simulink model "BlueBird_Formation"  (R2014a)
settings: Solver=FixedStepDiscrete  StartTime=0.0  StopTime=inf  FixedStep=0.033  RelTol=1e-3
undefined symbols (not defined in the file or in its folder): BlueBird_uni_todiff, simiam, Z_Ref
libraries: KSim x4
settings Model: SnapshotBufferSize=100  Creator=jdelacroix  LastModifiedBy=Bird
settings DataIOCC: SignalLoggingSaveFormat=ModelDataLogs
settings OptimizationCC: ExpressionDepthLimit=2147483647
settings DebuggingCC: UnderspecifiedInitializationDetection=Classic  FcnCallInpInsideContextMsg=EnableAllAsWarning  StateNameClashWarn=warning

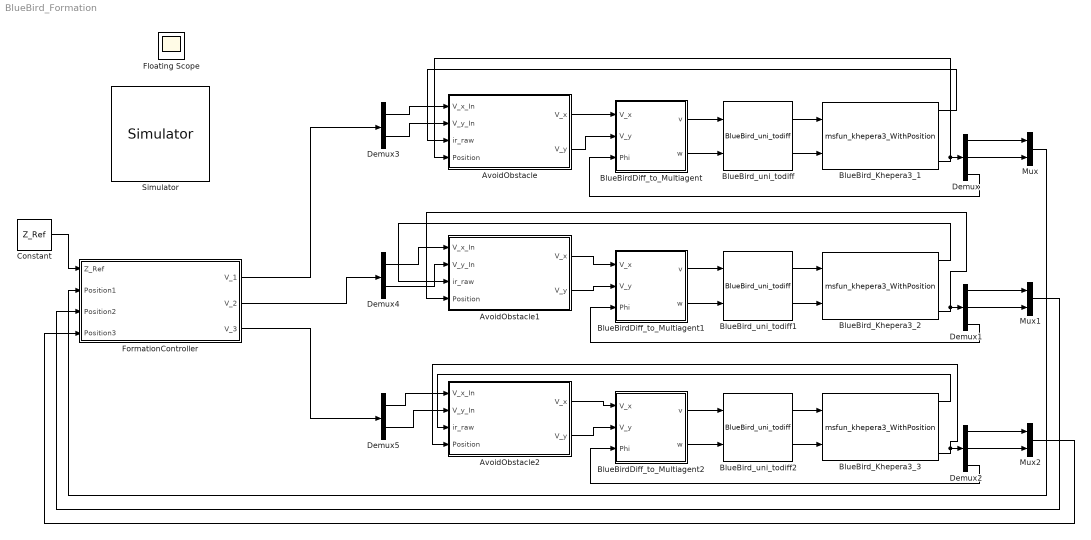
== system BlueBird_Formation ==
  AvoidObstacle : MATLAB Function  TreatAsAtomicUnit=on
  AvoidObstacle1 : MATLAB Function  TreatAsAtomicUnit=on
  AvoidObstacle2 : MATLAB Function  TreatAsAtomicUnit=on
  BlueBirdDiff_to_Multiagent : Subsystem  AncestorBlock=simiam/BlueBird_uni_todiff  mask(BlueBird_uni_todiff){l=2}
      mask prompts: l "偏移量（cm）"
      mask help: 这个模块完成自行车模型向机器人模型的转换。
  BlueBirdDiff_to_Multiagent1 : Subsystem  AncestorBlock=simiam/BlueBird_uni_todiff  mask(BlueBird_uni_todiff){l=2}
      mask prompts: l "偏移量（cm）"
      mask help: 这个模块完成自行车模型向机器人模型的转换。
  BlueBirdDiff_to_Multiagent2 : Subsystem  AncestorBlock=simiam/BlueBird_uni_todiff  mask(BlueBird_uni_todiff){l=2}
      mask prompts: l "偏移量（cm）"
      mask help: 这个模块完成自行车模型向机器人模型的转换。
  BlueBird_Khepera3_1 : M-S-Function  AncestorBlock=simiam/Khepera III  FunctionName=msfun_khepera3_WithPosition  Parameters=x_0,y_0,theta_0,ShowObservation  mask(Khepera3){x_0=0, y_0=0, theta_0=0, robot_id=1, ShowObservation=off}
      mask prompts: robot_id "ID"; ShowObservation "显示观测"
      mask Display:
      | port_label('output', 1, 'ir_raw')
      | port_label('output', 2, 'wheel_ticks')
      | port_label('output', 3, 'PosFromSim')
      | port_label('output', 4, 'EKF_Out')
      | 
      | port_label('input', 1, 'vel_r')
      | port_label('input', 2, 'vel_l')
  BlueBird_Khepera3_2 : M-S-Function  AncestorBlock=simiam/Khepera III  FunctionName=msfun_khepera3_WithPosition  Parameters=x_0,y_0,theta_0,ShowObservation  mask(Khepera3){x_0=-0.8, y_0=0, theta_0=-pi/2, robot_id=2, ShowObservation=off}
      mask prompts: robot_id "ID"; ShowObservation "显示观测"
      mask Display:
      | port_label('output', 1, 'ir_raw')
      | port_label('output', 2, 'wheel_ticks')
      | port_label('output', 3, 'PosFromSim')
      | port_label('output', 4, 'EKF_Out')
      | 
      | port_label('input', 1, 'vel_r')
      | port_label('input', 2, 'vel_l')
  BlueBird_Khepera3_3 : M-S-Function  AncestorBlock=simiam/Khepera III  FunctionName=msfun_khepera3_WithPosition  Parameters=x_0,y_0,theta_0,ShowObservation  mask(Khepera3){x_0=0.8, y_0=0, theta_0=pi/2, robot_id=3, ShowObservation=on}
      mask prompts: robot_id "ID"; ShowObservation "显示观测"
      mask Display:
      | port_label('output', 1, 'ir_raw')
      | port_label('output', 2, 'wheel_ticks')
      | port_label('output', 3, 'PosFromSim')
      | port_label('output', 4, 'EKF_Out')
      | 
      | port_label('input', 1, 'vel_r')
      | port_label('input', 2, 'vel_l')
  BlueBird_uni_todiff : KSim/BlueBird_uni_todiff  r_R=0.0213200003  r_L=0.0213200003  b=0.0896796882
  BlueBird_uni_todiff1 : KSim/BlueBird_uni_todiff  r_R=0.0213200003  r_L=0.0213200003  b=0.0896796882
  BlueBird_uni_todiff2 : KSim/BlueBird_uni_todiff  r_R=0.0213200003  r_L=0.0213200003  b=0.0896796882
  Constant : Constant  Value=Z_Ref
  Demux : Demux  Outputs=3
  Demux1 : Demux  Outputs=3
  Demux2 : Demux  Outputs=3
  Demux3 : Demux  Outputs=2
  Demux4 : Demux  Outputs=2
  Demux5 : Demux  Outputs=2
  FormationController : MATLAB Function  TreatAsAtomicUnit=on
  Mux : Mux  Inputs=2
  Mux1 : Mux  Inputs=2
  Mux2 : Mux  Inputs=2
  Simulator : KSim/Simulator  Priority=1
  Floating Scope : Scope
      settings: Floating=on
  wires:
  BlueBird_uni_todiff/1 -> BlueBird_Khepera3_1/1
  BlueBird_uni_todiff/2 -> BlueBird_Khepera3_1/2
  BlueBirdDiff_to_Multiagent/1(v) -> BlueBird_uni_todiff/1
  BlueBirdDiff_to_Multiagent/2(w) -> BlueBird_uni_todiff/2
  Demux/3 -> BlueBirdDiff_to_Multiagent/3(Phi)
  BlueBird_uni_todiff1/1 -> BlueBird_Khepera3_2/1
  BlueBird_uni_todiff1/2 -> BlueBird_Khepera3_2/2
  BlueBirdDiff_to_Multiagent1/1(v) -> BlueBird_uni_todiff1/1
  BlueBirdDiff_to_Multiagent1/2(w) -> BlueBird_uni_todiff1/2
  Demux1/3 -> BlueBirdDiff_to_Multiagent1/3(Phi)
  BlueBird_uni_todiff2/1 -> BlueBird_Khepera3_3/1
  BlueBird_uni_todiff2/2 -> BlueBird_Khepera3_3/2
  BlueBirdDiff_to_Multiagent2/1(v) -> BlueBird_uni_todiff2/1
  BlueBirdDiff_to_Multiagent2/2(w) -> BlueBird_uni_todiff2/2
  Demux2/3 -> BlueBirdDiff_to_Multiagent2/3(Phi)
  Constant/1 -> FormationController/1(Z_Ref)
  FormationController/1(V_1) -> Demux3/1
  FormationController/2(V_2) -> Demux4/1
  FormationController/3(V_3) -> Demux5/1
  Demux/1 -> Mux/1
  Demux/2 -> Mux/2
  Demux1/1 -> Mux1/1
  Demux1/2 -> Mux1/2
  Demux2/2 -> Mux2/2
  Demux2/1 -> Mux2/1
  Mux/1 -> FormationController/2(Position1)
  Mux1/1 -> FormationController/3(Position2)
  Mux2/1 -> FormationController/4(Position3)
  AvoidObstacle/1(V_x) -> BlueBirdDiff_to_Multiagent/1(V_x)
  Demux3/1 -> AvoidObstacle/1(V_x_In)
  AvoidObstacle/2(V_y) -> BlueBirdDiff_to_Multiagent/2(V_y)
  Demux3/2 -> AvoidObstacle/2(V_y_In)
  BlueBird_Khepera3_1/1 -> AvoidObstacle/3(ir_raw)
  AvoidObstacle1/1(V_x) -> BlueBirdDiff_to_Multiagent1/1(V_x)
  AvoidObstacle1/2(V_y) -> BlueBirdDiff_to_Multiagent1/2(V_y)
  AvoidObstacle2/1(V_x) -> BlueBirdDiff_to_Multiagent2/1(V_x)
  AvoidObstacle2/2(V_y) -> BlueBirdDiff_to_Multiagent2/2(V_y)
  Demux4/1 -> AvoidObstacle1/1(V_x_In)
  Demux4/2 -> AvoidObstacle1/2(V_y_In)
  Demux5/1 -> AvoidObstacle2/1(V_x_In)
  Demux5/2 -> AvoidObstacle2/2(V_y_In)
  BlueBird_Khepera3_2/1 -> AvoidObstacle1/3(ir_raw)
  BlueBird_Khepera3_3/1 -> AvoidObstacle2/3(ir_raw)
  BlueBird_Khepera3_1/4 -> AvoidObstacle/4(Position), Demux/1
  BlueBird_Khepera3_2/4 -> AvoidObstacle1/4(Position), Demux1/1
  BlueBird_Khepera3_3/4 -> AvoidObstacle2/4(Position), Demux2/1

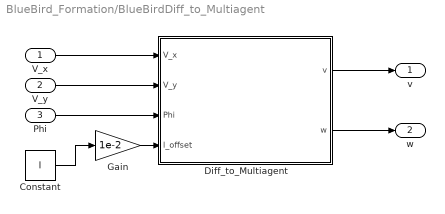
== system BlueBird_Formation/BlueBirdDiff_to_Multiagent ==
  V_x : Inport
  V_y : Inport  Port=2
  Phi : Inport  Port=3
  Constant : Constant  Value=l
  Diff_to_Multiagent : MATLAB Function  TreatAsAtomicUnit=on
  Gain : Gain  Gain=1e-2
  v : Outport
  w : Outport  Port=2
  wires:
  V_x/1 -> Diff_to_Multiagent/1(V_x)
  V_y/1 -> Diff_to_Multiagent/2(V_y)
  Phi/1 -> Diff_to_Multiagent/3(Phi)
  Constant/1 -> Gain/1
  Gain/1 -> Diff_to_Multiagent/4(l_offset)
  Diff_to_Multiagent/1(v) -> v/1
  Diff_to_Multiagent/2(w) -> w/1

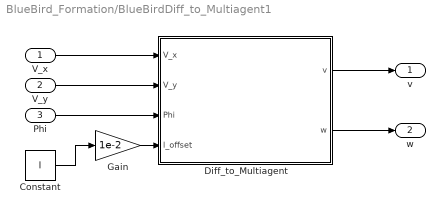
== system BlueBird_Formation/BlueBirdDiff_to_Multiagent1 ==
  V_x : Inport
  V_y : Inport  Port=2
  Phi : Inport  Port=3
  Constant : Constant  Value=l
  Diff_to_Multiagent : MATLAB Function  TreatAsAtomicUnit=on
  Gain : Gain  Gain=1e-2
  v : Outport
  w : Outport  Port=2
  wires:
  V_x/1 -> Diff_to_Multiagent/1(V_x)
  V_y/1 -> Diff_to_Multiagent/2(V_y)
  Phi/1 -> Diff_to_Multiagent/3(Phi)
  Constant/1 -> Gain/1
  Gain/1 -> Diff_to_Multiagent/4(l_offset)
  Diff_to_Multiagent/1(v) -> v/1
  Diff_to_Multiagent/2(w) -> w/1

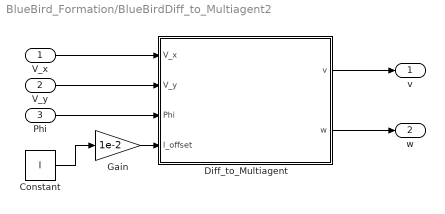
== system BlueBird_Formation/BlueBirdDiff_to_Multiagent2 ==
  V_x : Inport
  V_y : Inport  Port=2
  Phi : Inport  Port=3
  Constant : Constant  Value=l
  Diff_to_Multiagent : MATLAB Function  TreatAsAtomicUnit=on
  Gain : Gain  Gain=1e-2
  v : Outport
  w : Outport  Port=2
  wires:
  V_x/1 -> Diff_to_Multiagent/1(V_x)
  V_y/1 -> Diff_to_Multiagent/2(V_y)
  Phi/1 -> Diff_to_Multiagent/3(Phi)
  Constant/1 -> Gain/1
  Gain/1 -> Diff_to_Multiagent/4(l_offset)
  Diff_to_Multiagent/1(v) -> v/1
  Diff_to_Multiagent/2(w) -> w/1

== matlab function BlueBird_Formation/BlueBirdDiff_to_Multiagent1/Diff_to_Multiagent ==
  data: V_x input; V_y input; v output; Phi input; l_offset input; w output
function [v,w] = BlueBird_Diff_to_Multiagent(V_x,V_y,Phi,l_offset)
%#codegen
%l_offset在这个函数里是米
if(l_offset >0)
    Temp = [1 0 ; 0 1/l_offset]*[cos(-Phi) -sin(-Phi); sin(-Phi) cos(-Phi)]*[V_x ; V_y];
    v = Temp(1,1);
    w = Temp(2,1);
else
    v = 0;
    w = 0;
end

== matlab function BlueBird_Formation/BlueBirdDiff_to_Multiagent/Diff_to_Multiagent ==
  data: V_x input; V_y input; v output; Phi input; l_offset input; w output
function [v,w] = BlueBird_Diff_to_Multiagent(V_x,V_y,Phi,l_offset)
%#codegen
%l_offset在这个函数里是米
if(l_offset >0)
    Temp = [1 0 ; 0 1/l_offset]*[cos(-Phi) -sin(-Phi); sin(-Phi) cos(-Phi)]*[V_x ; V_y];
    v = Temp(1,1);
    w = Temp(2,1);
else
    v = 0;
    w = 0;
end

== matlab function BlueBird_Formation/BlueBirdDiff_to_Multiagent2/Diff_to_Multiagent ==
  data: V_x input; V_y input; v output; Phi input; l_offset input; w output
function [v,w] = BlueBird_Diff_to_Multiagent(V_x,V_y,Phi,l_offset)
%#codegen
%l_offset在这个函数里是米
if(l_offset >0)
    Temp = [1 0 ; 0 1/l_offset]*[cos(-Phi) -sin(-Phi); sin(-Phi) cos(-Phi)]*[V_x ; V_y];
    v = Temp(1,1);
    w = Temp(2,1);
else
    v = 0;
    w = 0;
end

== matlab function BlueBird_Formation/FormationController ==
  data: Z_Ref input; V_1 output; Position1 input; Position2 input; Position3 input; V_2 output; V_3 output
function [V_1,V_2,V_3] = FormationController(Z_Ref,Position1,Position2,Position3)
%#codegen
k = 0.5;%速度调节参数

D_Conv = [1 0 ; -1 1 ; 0 -1]; %表示链接关系
Eye_Matrix = eye(2); % 处理二维
D = kron(D_Conv,Eye_Matrix);

x = [Position1 ; Position2 ; Position3];%机器人的位置向量
z = D' * x;
e = Z_Ref - z;

u = k * D * e;


V_1 = u(1:2,1);
V_2 = u(3:4,1);
V_3 = u(5:6,1);

== matlab function BlueBird_Formation/AvoidObstacle ==
  data: V_x_In input; V_x output; V_y_In input; V_y output; ir_raw input; Position input
function [V_x,V_y] = AvoidObstacle_Speed(V_x_In,V_y_In,ir_raw,Position)
%#codegen
persistent Counter
if isempty(Counter)
    Counter = 0;
end

%没有噪声的前提下，将原始红外数据转换为距离
    [ir_distances,ObstacleDetected] = IR_Raw_to_Distances(ir_raw);
    if(ObstacleDetected > 0)
        IF_Obstacle = 1;
        Counter = 25;
    end
    
    if(Counter > 0)
        IF_Obstacle = 1;
        Counter = Counter - 1;
    else
        IF_Obstacle = -1;
    end
    
    if(IF_Obstacle > 0)

        %由于红外传感器在x正轴方向安装的比负方向多，将传感器9的数值+一点，加以修正
        FixIR_9_Number = 0.364;%应该补偿0.3642，现在少补偿一点，让平时，机器人的向量决策为当前机器人的前方
        ir_distances = ir_distances + ([0 0 0 0 0 0 0 0 1]')*FixIR_9_Number;

        %利用红外距离数据计算以机器人坐标的周围物体：
        Obstacle_AroundRobot = zeros(3,9);

        for i = 1:1:9%一共有九个红外
             IR_Position_I = GetIR_Position(i);
             IR_Transformation_Matrix_I = Transformation_Matrix(IR_Position_I(1,1),IR_Position_I(2,1),IR_Position_I(3,1));
             Obstacle_AroundRobot_I = IR_Transformation_Matrix_I*[ir_distances(i) ; 0 ; 1];

             Obstacle_AroundRobot(:,i) = Obstacle_AroundRobot_I;
        end
        %将以机器人为原点的周围障碍物信息转换为以世界坐标系的信息
        Obstacle_AroundRobot_World = Transformation_Matrix(Position(1,1), Position(2,1), Position(3,1))*Obstacle_AroundRobot;
        ObstaclesSpeed = AvoidObstacles_NextPoint(Obstacle_AroundRobot_World,Position);
        V_x = ObstaclesSpeed(1,1);
        V_y = ObstaclesSpeed(2,1);

    else
        V_x = V_x_In;
        V_y = V_y_In;
    end

end

function [Answer,ObstacleDetected] = IR_Raw_to_Distances(ir_raw)
    %将传感器数据转换为距离
    %reallog就是以e为底的对数
    SafeNumber = 150;
    MaxNumber = 3960;
    
    ir_raw_Internal = ir_raw;
    
    %处理掉ir_raw_Internal里面<SafeNumber的数值
    Number_List = find(ir_raw_Internal < SafeNumber);
    ir_raw_Internal(Number_List) = SafeNumber;
    
    %找到检出障碍物的传感器在Answer中的位置
    ObstacleDetected = find(ir_raw_Internal > SafeNumber);
    ObstacleDetected = length(ObstacleDetected);
    
    %处理掉超过允许最大值的值
    Number_List = find(ir_raw_Internal > MaxNumber);
    ir_raw_Internal(Number_List) = MaxNumber;
    
    
    Answer = 0.02-reallog(ir_raw_Internal/3960)/30;
end

function [Answer] = GetIR_Position(IR_Number)
    Pose2D_Use = simiam.ui.Pose2D(0,0,0);
    IR_Position = [
        -0.038  0.049 Pose2D_Use.deg2rad(128);
        0.017  0.063  Pose2D_Use.deg2rad(75);
        0.051  0.045  Pose2D_Use.deg2rad(42);
        0.067  0.015  Pose2D_Use.deg2rad(13);
        0.067  -0.015  Pose2D_Use.deg2rad(-13);
        0.051  -0.045  Pose2D_Use.deg2rad(-42);
        0.017  -0.063  Pose2D_Use.deg2rad(-75);
        -0.038  -0.049  Pose2D_Use.deg2rad(-128);
        -0.052  0.000  Pose2D_Use.deg2rad(180)
    ];
    Answer = (IR_Position(IR_Number,:))';
    %Answer = 0;
end

function [Answer] = Transformation_Matrix(x, y, theta)
    %坐标转移矩阵
    AvoidObstacles_Use = simiam.controller.AvoidObstacles();
    Answer = AvoidObstacles_Use.get_transformation_matrix(x, y, theta);
end

function [ObstaclesSpeed] = AvoidObstacles_NextPoint(Obstacle_AroundRobot_World,Position)
FixIR_9_Number = 0.364;

%障碍物坐标向量权重
sensor_gains = [1 1 1 1 1 1 1 1 1];
%(ir_distances_rf-repmat([x;y],1,9))这个是以机器人为起点，以障碍物为终点的向量列
%去掉Obstacle_AroundRobot_World里面的最后一行1
ir_distances_rf = Obstacle_AroundRobot_World(1:2,:);
u_i = (ir_distances_rf-repmat([Position(1,1);Position(2,1)],1,9))*diag(sensor_gains);
%u_i是给每一个障碍物向量加一个权重，正如说明书上写的
%然后把这些向量加起来,得到最不可能有障碍物方向的向量
SumOfObstacleVector_Word = sum(u_i,2);
NextAngle = atan2(SumOfObstacleVector_Word(2,1),SumOfObstacleVector_Word(1,1));

k = 0.1;
ObstaclesSpeed = k*[cos(NextAngle) ; sin(NextAngle)];
end

== matlab function BlueBird_Formation/AvoidObstacle1 ==
  data: V_x_In input; V_x output; V_y_In input; V_y output; ir_raw input; Position input
function [V_x,V_y] = AvoidObstacle_Speed(V_x_In,V_y_In,ir_raw,Position)
%#codegen
persistent Counter
if isempty(Counter)
    Counter = 0;
end

%没有噪声的前提下，将原始红外数据转换为距离
    [ir_distances,ObstacleDetected] = IR_Raw_to_Distances(ir_raw);
    if(ObstacleDetected > 0)
        IF_Obstacle = 1;
        Counter = 25;
    end
    
    if(Counter > 0)
        IF_Obstacle = 1;
        Counter = Counter - 1;
    else
        IF_Obstacle = -1;
    end
    
    if(IF_Obstacle > 0)

        %由于红外传感器在x正轴方向安装的比负方向多，将传感器9的数值+一点，加以修正
        FixIR_9_Number = 0.364;%应该补偿0.3642，现在少补偿一点，让平时，机器人的向量决策为当前机器人的前方
        ir_distances = ir_distances + ([0 0 0 0 0 0 0 0 1]')*FixIR_9_Number;

        %利用红外距离数据计算以机器人坐标的周围物体：
        Obstacle_AroundRobot = zeros(3,9);

        for i = 1:1:9%一共有九个红外
             IR_Position_I = GetIR_Position(i);
             IR_Transformation_Matrix_I = Transformation_Matrix(IR_Position_I(1,1),IR_Position_I(2,1),IR_Position_I(3,1));
             Obstacle_AroundRobot_I = IR_Transformation_Matrix_I*[ir_distances(i) ; 0 ; 1];

             Obstacle_AroundRobot(:,i) = Obstacle_AroundRobot_I;
        end
        %将以机器人为原点的周围障碍物信息转换为以世界坐标系的信息
        Obstacle_AroundRobot_World = Transformation_Matrix(Position(1,1), Position(2,1), Position(3,1))*Obstacle_AroundRobot;
        ObstaclesSpeed = AvoidObstacles_NextPoint(Obstacle_AroundRobot_World,Position);
        V_x = ObstaclesSpeed(1,1);
        V_y = ObstaclesSpeed(2,1);

    else
        V_x = V_x_In;
        V_y = V_y_In;
    end

end

function [Answer,ObstacleDetected] = IR_Raw_to_Distances(ir_raw)
    %将传感器数据转换为距离
    %reallog就是以e为底的对数
    SafeNumber = 150;
    MaxNumber = 3960;
    
    ir_raw_Internal = ir_raw;
    
    %处理掉ir_raw_Internal里面<SafeNumber的数值
    Number_List = find(ir_raw_Internal < SafeNumber);
    ir_raw_Internal(Number_List) = SafeNumber;
    
    %找到检出障碍物的传感器在Answer中的位置
    ObstacleDetected = find(ir_raw_Internal > SafeNumber);
    ObstacleDetected = length(ObstacleDetected);
    
    %处理掉超过允许最大值的值
    Number_List = find(ir_raw_Internal > MaxNumber);
    ir_raw_Internal(Number_List) = MaxNumber;
    
    
    Answer = 0.02-reallog(ir_raw_Internal/3960)/30;
end

function [Answer] = GetIR_Position(IR_Number)
    Pose2D_Use = simiam.ui.Pose2D(0,0,0);
    IR_Position = [
        -0.038  0.049 Pose2D_Use.deg2rad(128);
        0.017  0.063  Pose2D_Use.deg2rad(75);
        0.051  0.045  Pose2D_Use.deg2rad(42);
        0.067  0.015  Pose2D_Use.deg2rad(13);
        0.067  -0.015  Pose2D_Use.deg2rad(-13);
        0.051  -0.045  Pose2D_Use.deg2rad(-42);
        0.017  -0.063  Pose2D_Use.deg2rad(-75);
        -0.038  -0.049  Pose2D_Use.deg2rad(-128);
        -0.052  0.000  Pose2D_Use.deg2rad(180)
    ];
    Answer = (IR_Position(IR_Number,:))';
    %Answer = 0;
end

function [Answer] = Transformation_Matrix(x, y, theta)
    %坐标转移矩阵
    AvoidObstacles_Use = simiam.controller.AvoidObstacles();
    Answer = AvoidObstacles_Use.get_transformation_matrix(x, y, theta);
end

function [ObstaclesSpeed] = AvoidObstacles_NextPoint(Obstacle_AroundRobot_World,Position)
FixIR_9_Number = 0.364;

%障碍物坐标向量权重
sensor_gains = [1 1 1 1 1 1 1 1 1];
%(ir_distances_rf-repmat([x;y],1,9))这个是以机器人为起点，以障碍物为终点的向量列
%去掉Obstacle_AroundRobot_World里面的最后一行1
ir_distances_rf = Obstacle_AroundRobot_World(1:2,:);
u_i = (ir_distances_rf-repmat([Position(1,1);Position(2,1)],1,9))*diag(sensor_gains);
%u_i是给每一个障碍物向量加一个权重，正如说明书上写的
%然后把这些向量加起来,得到最不可能有障碍物方向的向量
SumOfObstacleVector_Word = sum(u_i,2);
NextAngle = atan2(SumOfObstacleVector_Word(2,1),SumOfObstacleVector_Word(1,1));

k = 0.1;
ObstaclesSpeed = k*[cos(NextAngle) ; sin(NextAngle)];
end

== matlab function BlueBird_Formation/AvoidObstacle2 ==
  data: V_x_In input; V_x output; V_y_In input; V_y output; ir_raw input; Position input
function [V_x,V_y] = AvoidObstacle_Speed(V_x_In,V_y_In,ir_raw,Position)
%#codegen
persistent Counter
if isempty(Counter)
    Counter = 0;
end

%没有噪声的前提下，将原始红外数据转换为距离
    [ir_distances,ObstacleDetected] = IR_Raw_to_Distances(ir_raw);
    if(ObstacleDetected > 0)
        IF_Obstacle = 1;
        Counter = 25;
    end
    
    if(Counter > 0)
        IF_Obstacle = 1;
        Counter = Counter - 1;
    else
        IF_Obstacle = -1;
    end
    
    if(IF_Obstacle > 0)

        %由于红外传感器在x正轴方向安装的比负方向多，将传感器9的数值+一点，加以修正
        FixIR_9_Number = 0.364;%应该补偿0.3642，现在少补偿一点，让平时，机器人的向量决策为当前机器人的前方
        ir_distances = ir_distances + ([0 0 0 0 0 0 0 0 1]')*FixIR_9_Number;

        %利用红外距离数据计算以机器人坐标的周围物体：
        Obstacle_AroundRobot = zeros(3,9);

        for i = 1:1:9%一共有九个红外
             IR_Position_I = GetIR_Position(i);
             IR_Transformation_Matrix_I = Transformation_Matrix(IR_Position_I(1,1),IR_Position_I(2,1),IR_Position_I(3,1));
             Obstacle_AroundRobot_I = IR_Transformation_Matrix_I*[ir_distances(i) ; 0 ; 1];

             Obstacle_AroundRobot(:,i) = Obstacle_AroundRobot_I;
        end
        %将以机器人为原点的周围障碍物信息转换为以世界坐标系的信息
        Obstacle_AroundRobot_World = Transformation_Matrix(Position(1,1), Position(2,1), Position(3,1))*Obstacle_AroundRobot;
        ObstaclesSpeed = AvoidObstacles_NextPoint(Obstacle_AroundRobot_World,Position);
        V_x = ObstaclesSpeed(1,1);
        V_y = ObstaclesSpeed(2,1);

    else
        V_x = V_x_In;
        V_y = V_y_In;
    end

end

function [Answer,ObstacleDetected] = IR_Raw_to_Distances(ir_raw)
    %将传感器数据转换为距离
    %reallog就是以e为底的对数
    SafeNumber = 150;
    MaxNumber = 3960;
    
    ir_raw_Internal = ir_raw;
    
    %处理掉ir_raw_Internal里面<SafeNumber的数值
    Number_List = find(ir_raw_Internal < SafeNumber);
    ir_raw_Internal(Number_List) = SafeNumber;
    
    %找到检出障碍物的传感器在Answer中的位置
    ObstacleDetected = find(ir_raw_Internal > SafeNumber);
    ObstacleDetected = length(ObstacleDetected);
    
    %处理掉超过允许最大值的值
    Number_List = find(ir_raw_Internal > MaxNumber);
    ir_raw_Internal(Number_List) = MaxNumber;
    
    
    Answer = 0.02-reallog(ir_raw_Internal/3960)/30;
end

function [Answer] = GetIR_Position(IR_Number)
    Pose2D_Use = simiam.ui.Pose2D(0,0,0);
    IR_Position = [
        -0.038  0.049 Pose2D_Use.deg2rad(128);
        0.017  0.063  Pose2D_Use.deg2rad(75);
        0.051  0.045  Pose2D_Use.deg2rad(42);
        0.067  0.015  Pose2D_Use.deg2rad(13);
        0.067  -0.015  Pose2D_Use.deg2rad(-13);
        0.051  -0.045  Pose2D_Use.deg2rad(-42);
        0.017  -0.063  Pose2D_Use.deg2rad(-75);
        -0.038  -0.049  Pose2D_Use.deg2rad(-128);
        -0.052  0.000  Pose2D_Use.deg2rad(180)
    ];
    Answer = (IR_Position(IR_Number,:))';
    %Answer = 0;
end

function [Answer] = Transformation_Matrix(x, y, theta)
    %坐标转移矩阵
    AvoidObstacles_Use = simiam.controller.AvoidObstacles();
    Answer = AvoidObstacles_Use.get_transformation_matrix(x, y, theta);
end

function [ObstaclesSpeed] = AvoidObstacles_NextPoint(Obstacle_AroundRobot_World,Position)
FixIR_9_Number = 0.364;

%障碍物坐标向量权重
sensor_gains = [1 1 1 1 1 1 1 1 1];
%(ir_distances_rf-repmat([x;y],1,9))这个是以机器人为起点，以障碍物为终点的向量列
%去掉Obstacle_AroundRobot_World里面的最后一行1
ir_distances_rf = Obstacle_AroundRobot_World(1:2,:);
u_i = (ir_distances_rf-repmat([Position(1,1);Position(2,1)],1,9))*diag(sensor_gains);
%u_i是给每一个障碍物向量加一个权重，正如说明书上写的
%然后把这些向量加起来,得到最不可能有障碍物方向的向量
SumOfObstacleVector_Word = sum(u_i,2);
NextAngle = atan2(SumOfObstacleVector_Word(2,1),SumOfObstacleVector_Word(1,1));

k = 0.1;
ObstaclesSpeed = k*[cos(NextAngle) ; sin(NextAngle)];
end
